simulink model "get_SEA_pos"  (R2016b)
settings: Solver=VariableStepAuto  StartTime=0.0  StopTime=0  RelTol=1e-3
undefined symbols (not defined in the file or in its folder): Earth, gps_sec, gps_week, sc_alt, UW_lat_lon, WGS84
libraries: aerolibtransform2 x1, time_coord_rotation_lib x1
settings Model: Creator=Taylor  LastModifiedBy=Taylor

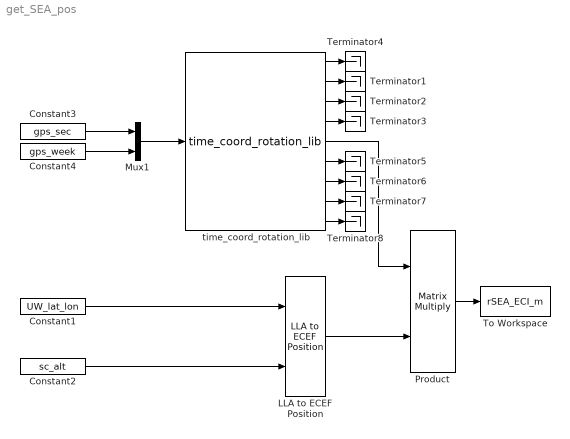
== system get_SEA_pos ==
  Constant1 : Constant  Value=UW_lat_lon
  Constant2 : Constant  Value=sc_alt
  Constant3 : Constant  Value=gps_sec
  Constant4 : Constant  Value=gps_week
  LLA to ECEF Position : aerolibtransform2/LLA to ECEF Position  units=Metric (MKS)  ptype=Earth (WGS84)  F=1/298.257223563  R=6378137
  Mux1 : Mux  Inputs=2
  Product : Product  Multiplication=Matrix(*)
  Terminator{1..8} (8 alike) : Terminator
  To Workspace : ToWorkspace  VariableName=rSEA_ECI_m  SampleTime=-1
  time_coord_rotation_lib : time_coord_rotation_lib/time_coord_rotation_lib
  wires:
  Constant2/1 -> LLA to ECEF Position/2
  Constant1/1 -> LLA to ECEF Position/1
  LLA to ECEF Position/1 -> Product/2
  time_coord_rotation_lib/5 -> Product/1
  Product/1 -> To Workspace/1
  Mux1/1 -> time_coord_rotation_lib/1
  Constant3/1 -> Mux1/1
  Constant4/1 -> Mux1/2
  time_coord_rotation_lib/1 -> Terminator4/1
  time_coord_rotation_lib/2 -> Terminator1/1
  time_coord_rotation_lib/3 -> Terminator2/1
  time_coord_rotation_lib/4 -> Terminator3/1
  time_coord_rotation_lib/6 -> Terminator5/1
  time_coord_rotation_lib/7 -> Terminator6/1
  time_coord_rotation_lib/8 -> Terminator7/1
  time_coord_rotation_lib/9 -> Terminator8/1
